simulink model "top10x20"  (Simulink 6.3)
settings: Solver=FixedStepDiscrete  StartTime=0.0  StopTime=3000  FixedStep=1  RelTol=1e-3
PreLoadFcn:
  | disp('Convolutional Interleaver 10x20')
  | disp(' 10 Branches')
  | disp(' FifoDepth = 20')
  | 
  | FifoDepth=20;
  | SymbolWidth = 8;
InitFcn:
  | %% DSPBuilder Start
  | alt_dspbuilder_update_model(bdroot)
  | %% DSPBuilder End
libraries: allblocks_alteradspbuilder2 x72, simulink x1
settings Model: LastModifiedBy=LKONG  StrictBusMsg=None
settings OptimizationCC: BooleanDataType=off  InlineInvariantSignals=on
settings DebuggingCC: SolverPrmCheckMsg=none
settings HardwareCC: TargetUnknown=on

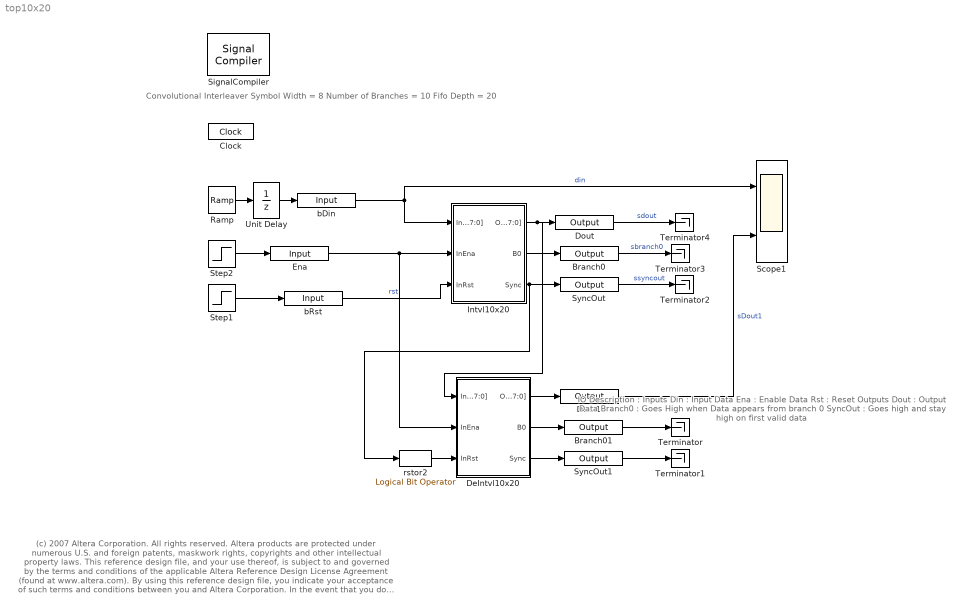
== system top10x20 ==
  note: (c) 2007 Altera Corporation. All rights reserved.  Altera products are protected under numerous U.S. and foreign patents, maskwork rights, copyrights and other intellectual property laws.
      | This reference design file, and your use thereof, is subject to and governed by the terms and conditions of the applicable Altera Reference Design License Agreement (found at www.altera.com).
      | By using this reference design file, you indicate your acceptance of such terms and conditions between you and Altera Corporation.
      | In the event that you do not agree with such terms and conditions, you may not use the reference design file and please promptly destroy any copies you have made.
      | This reference design file being provided on an "as-is" basis and as an accommodation and therefore all warranties, representations or guarantees of any kind (whether express, implied or statutory)
      | including, without limitation, warranties of merchantability, non-infringement, or fitness for a particular purpose, are specifically disclaimed.
      | By making this reference design file available, Altera expressly does not recommend, suggest or require that this reference design file be used in combination with any other product not provided by Altera
  note: IO Description :
      |
      | Inputs
      |            Din    : Input Data
      |            Ena   : Enable Data
      |            Rst    : Reset
      |
      | Outputs
      |           Dout        : Output Data
      |           Branch0 : Goes High when Data appears from branch 0
      |           SyncOut : Goes high and stay high on first valid data
  note: Convolutional Interleaver
      | Symbol Width = 8
      | Number of Branches = 10
      | Fifo Depth = 20
  Branch0 : allblocks_alteradspbuilder2/Output  iofile=d:\wsTrunk\workspace\Documentation\DesignExamples\Demos\Transforms\CrossInterleaver12x17\tb_top10x20\top10x20_Branch0.capture  BusType=Single Bit  bwl=1  bwr=0  PORTTYPE=Output
  Branch01 : allblocks_alteradspbuilder2/Output  iofile=d:\wsTrunk\workspace\Documentation\DesignExamples\Demos\Transforms\CrossInterleaver12x17\tb_top10x20\top10x20_Branch01.capture  BusType=Single Bit  bwl=1  bwr=0  PORTTYPE=Output
  Clock : allblocks_alteradspbuilder2/Clock  ClockPeriod=100  ClockPeriodUnit=ns  SampleTime=1  SimulationStartCycle=5  PhaseOffset=0  Reset=aclr  ResetType=Active Low  Export=off
  DeIntvl10x20 : Subsystem  AncestorBlock=ALTELINK/AltLab/HDL SubSystem
      mask Type: SubSystem AlteraBlockSet
  Dout : allblocks_alteradspbuilder2/Output  iofile=d:\wsTrunk\workspace\Documentation\DesignExamples\Demos\Transforms\CrossInterleaver12x17\tb_top10x20\top10x20_Dout.capture  BusType=Signed Integer  bwl=8  bwr=0  PORTTYPE=Output
  Dout1 : allblocks_alteradspbuilder2/Output  iofile=d:\wsTrunk\workspace\Documentation\DesignExamples\Demos\Transforms\CrossInterleaver12x17\tb_top10x20\top10x20_Dout1.capture  BusType=Signed Integer  bwl=8  bwr=0  PORTTYPE=Output
  Ena : allblocks_alteradspbuilder2/Input  iofile=d:\wsTrunk\workspace\Documentation\DesignExamples\Demos\Transforms\CrossInterleaver12x17\tb_top10x20\top10x20_Ena.salt  BusType=Single Bit  bwl=1  bwr=0  SpecifyClock=off  PORTTYPE=Input
  Intvl10x20 : Subsystem  AncestorBlock=ALTELINK/AltLab/HDL SubSystem
      mask Type: SubSystem AlteraBlockSet
  Ramp : simulink/Sources/Ramp  slope=1  start=0  X0=3
  Scope1 : Scope  NumInputPorts=2
      settings: YMin=-5~-5  YMax=5~5
  SignalCompiler : allblocks_alteradspbuilder2/Signal Compiler  DeviceFamily=Cyclone IV GX  DeviceName=AUTO  EnableSignalTap=off  SignalTapDepth=128  UseBoardBlock=off  StpUseDefaultClock=on  StpClock=Clock
  Step1 : Step  Time=3  Before=1  After=0  SampleTime=1
  Step2 : Step  SampleTime=1
  SyncOut : allblocks_alteradspbuilder2/Output  iofile=d:\wsTrunk\workspace\Documentation\DesignExamples\Demos\Transforms\CrossInterleaver12x17\tb_top10x20\top10x20_SyncOut.capture  BusType=Single Bit  bwl=1  bwr=0  PORTTYPE=Output
  SyncOut1 : allblocks_alteradspbuilder2/Output  iofile=d:\wsTrunk\workspace\Documentation\DesignExamples\Demos\Transforms\CrossInterleaver12x17\tb_top10x20\top10x20_SyncOut1.capture  BusType=Single Bit  bwl=1  bwr=0  PORTTYPE=Output
  Terminator{,1..4} (5 alike) : Terminator
  Unit Delay : UnitDelay
  bDin : allblocks_alteradspbuilder2/Input  iofile=d:\wsTrunk\workspace\Documentation\DesignExamples\Demos\Transforms\CrossInterleaver12x17\tb_top10x20\top10x20_bDin.salt  BusType=Signed Integer  bwl=8  bwr=0  SpecifyClock=off  PORTTYPE=Input
  bRst : allblocks_alteradspbuilder2/Input  iofile=d:\wsTrunk\workspace\Documentation\DesignExamples\Demos\Transforms\CrossInterleaver12x17\tb_top10x20\top10x20_bRst.salt  BusType=Single Bit  bwl=1  bwr=0  SpecifyClock=off  PORTTYPE=Input
  rstor2 : allblocks_alteradspbuilder2/Logical Bit Operator  LogicalOperator=NOT  user_inputs=2
  wires:
  Intvl10x20/1(Out1[7:0]) -> Dout/1, DeIntvl10x20/1(InDin[7:0])
  bDin/1 -> Scope1/1, Intvl10x20/1(InDin[7:0])  "din"
  Ena/1 -> DeIntvl10x20/2(InEna), Intvl10x20/2(InEna)
  bRst/1 -> Intvl10x20/3(InRst)  "rst"
  Ramp/1 -> Unit Delay/1
  Step1/1 -> bRst/1
  Step2/1 -> Ena/1
  Intvl10x20/2(B0) -> Branch0/1
  Intvl10x20/3(Sync) -> SyncOut/1, rstor2/1
  Unit Delay/1 -> bDin/1
  rstor2/1 -> DeIntvl10x20/3(InRst)
  DeIntvl10x20/1(Out1[7:0]) -> Dout1/1
  DeIntvl10x20/2(B0) -> Branch01/1
  DeIntvl10x20/3(Sync) -> SyncOut1/1
  Dout1/1 -> Scope1/2  "sDout1"
  Branch01/1 -> Terminator/1
  SyncOut1/1 -> Terminator1/1
  SyncOut/1 -> Terminator2/1  "ssyncout"
  Branch0/1 -> Terminator3/1  "sbranch0"
  Dout/1 -> Terminator4/1  "sdout"

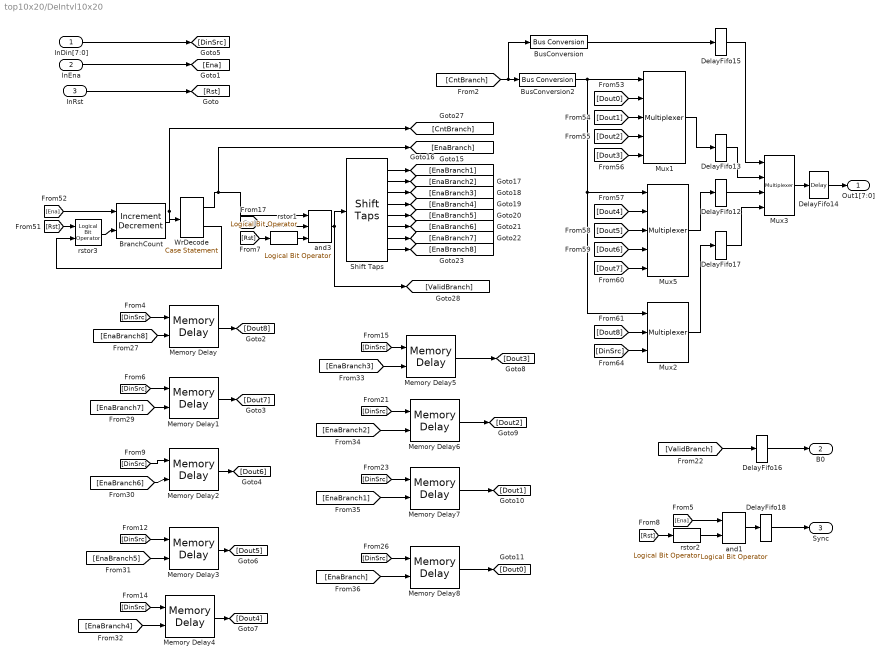
== system top10x20/DeIntvl10x20 ==
  InDin[7:0] : Inport
  InEna : Inport  Port=2
  InRst : Inport  Port=3
  BranchCount : allblocks_alteradspbuilder2/Increment Decrement  BusType=Unsigned Integer  bwl=4  bwr=0  SpecifyClock=off  clr_value=0  direction=Increment  phase_selection=1  use_ena=on  use_sclr=on
  BusConversion : allblocks_alteradspbuilder2/Bus Conversion  BusType=Unsigned Integer  ibwl=4  ibwr=0  bwl=2  bwr=0  bitToConnectToOutputLSB=2  round=off  saturate=off
  BusConversion2 : allblocks_alteradspbuilder2/Bus Conversion  BusType=Unsigned Integer  ibwl=4  ibwr=0  bwl=2  bwr=0  bitToConnectToOutputLSB=0  round=off  saturate=off
  DelayFifo{12..15,17} (5 alike) : allblocks_alteradspbuilder2/Delay  pipeline=1  ClockPhase=1  use_ena=off  use_sclr=off  use_init=off  reset_value=1
  DelayFifo16 : allblocks_alteradspbuilder2/Delay  pipeline=2  ClockPhase=1  use_ena=off  use_sclr=off  use_init=off  reset_value=1
  DelayFifo18 : allblocks_alteradspbuilder2/Delay  pipeline=2  ClockPhase=1  use_ena=off  use_sclr=off  use_init=off  reset_value=1
  Memory Delay : allblocks_alteradspbuilder2/Memory Delay  BusType=Inferred  bwl=8  bwr=0  pipeline=20  ram_type=AUTO  use_ena=on  use_sclr=off
  Memory Delay1 : allblocks_alteradspbuilder2/Memory Delay  BusType=Inferred  bwl=8  bwr=0  pipeline=40  ram_type=AUTO  use_ena=on  use_sclr=off
  Memory Delay2 : allblocks_alteradspbuilder2/Memory Delay  BusType=Inferred  bwl=8  bwr=0  pipeline=60  ram_type=AUTO  use_ena=on  use_sclr=off
  Memory Delay3 : allblocks_alteradspbuilder2/Memory Delay  BusType=Inferred  bwl=8  bwr=0  pipeline=80  ram_type=AUTO  use_ena=on  use_sclr=off
  Memory Delay4 : allblocks_alteradspbuilder2/Memory Delay  BusType=Inferred  bwl=8  bwr=0  pipeline=100  ram_type=AUTO  use_ena=on  use_sclr=off
  Memory Delay5 : allblocks_alteradspbuilder2/Memory Delay  BusType=Inferred  bwl=8  bwr=0  pipeline=120  ram_type=AUTO  use_ena=on  use_sclr=off
  Memory Delay6 : allblocks_alteradspbuilder2/Memory Delay  BusType=Inferred  bwl=8  bwr=0  pipeline=140  ram_type=AUTO  use_ena=on  use_sclr=off
  Memory Delay7 : allblocks_alteradspbuilder2/Memory Delay  BusType=Inferred  bwl=8  bwr=0  pipeline=160  ram_type=AUTO  use_ena=on  use_sclr=off
  Memory Delay8 : allblocks_alteradspbuilder2/Memory Delay  BusType=Inferred  bwl=8  bwr=0  pipeline=180  ram_type=AUTO  use_ena=on  use_sclr=off
  Mux1 : allblocks_alteradspbuilder2/Multiplexer  numInputs=4  pipeline=0  oneHot=off  use_ena=off  use_aclr=off
  Mux2 : allblocks_alteradspbuilder2/Multiplexer  numInputs=2  pipeline=0  oneHot=off  use_ena=off  use_aclr=off
  Mux3 : allblocks_alteradspbuilder2/Multiplexer  numInputs=3  pipeline=0  oneHot=off  use_ena=off  use_aclr=off
  Mux5 : allblocks_alteradspbuilder2/Multiplexer  numInputs=4  pipeline=0  oneHot=off  use_ena=off  use_aclr=off
  Shift Taps : allblocks_alteradspbuilder2/Shift Taps  number_of_taps=8  tap_distance=1  use_shiftout=off  use_ena=off  use_sclr=off  use_dedicated_circuitry=on  ram_type=AUTO
  WrDecode : allblocks_alteradspbuilder2/Case Statement  numOutputs=2  case_expression=0,9  formatted_case_expression=00000000,00001001  BusType=Signed Integer  bwl=8  bwr=0  pipeline=off  hasDefault=off
  and1 : allblocks_alteradspbuilder2/Logical Bit Operator  LogicalOperator=AND  user_inputs=2
  and3 : allblocks_alteradspbuilder2/Logical Bit Operator  LogicalOperator=AND  user_inputs=3
  rstor1 : allblocks_alteradspbuilder2/Logical Bit Operator  LogicalOperator=NOT  user_inputs=2
  rstor2 : allblocks_alteradspbuilder2/Logical Bit Operator  LogicalOperator=NOT  user_inputs=2
  rstor3 : allblocks_alteradspbuilder2/Logical Bit Operator  LogicalOperator=OR  user_inputs=2
  Out1[7:0] : Outport
  B0 : Outport  Port=2
  Sync : Outport  Port=3
  wires:
  and1/1 -> DelayFifo18/1
  rstor2/1 -> and1/2
  [Ena] -> and1/1
  [Rst] -> rstor2/1
  DelayFifo18/1 -> Sync/1
  BusConversion2/1 -> Mux2/1, Mux5/1, Mux1/1
  [CntBranch] -> BusConversion/1, BusConversion2/1
  Mux2/1 -> DelayFifo17/1
  Mux5/1 -> DelayFifo12/1
  DelayFifo17/1 -> Mux3/4
  DelayFifo12/1 -> Mux3/3
  Mux1/1 -> DelayFifo13/1
  DelayFifo16/1 -> B0/1
  [ValidBranch] -> DelayFifo16/1
  rstor1/1 -> and3/3
  [Ena] -> and3/2
  [Rst] -> rstor1/1
  and3/1 -> [ValidBranch], Shift Taps/1
  DelayFifo15/1 -> Mux3/1
  WrDecode/1 -> and3/1, [EnaBranch]
  DelayFifo13/1 -> Mux3/2
  [DinSrc] -> Mux2/3
  [Dout8] -> Mux2/2
  [Dout7] -> Mux5/5
  [Dout6] -> Mux5/4
  [Dout5] -> Mux5/3
  [Dout4] -> Mux5/2
  [Dout3] -> Mux1/5
  [Dout2] -> Mux1/4
  [Dout1] -> Mux1/3
  [Dout0] -> Mux1/2
  BusConversion/1 -> DelayFifo15/1
  Mux3/1 -> DelayFifo14/1
  Shift Taps/1 -> [EnaBranch1]
  Shift Taps/2 -> [EnaBranch2]
  Shift Taps/3 -> [EnaBranch3]
  Shift Taps/4 -> [EnaBranch4]
  Shift Taps/5 -> [EnaBranch5]
  Shift Taps/6 -> [EnaBranch6]
  Shift Taps/7 -> [EnaBranch7]
  Shift Taps/8 -> [EnaBranch8]
  [Ena] -> BranchCount/1
  [Rst] -> rstor3/1
  rstor3/1 -> BranchCount/2
  WrDecode/2 -> rstor3/2
  BranchCount/1 -> WrDecode/1, [CntBranch]
  DelayFifo14/1 -> Out1[7:0]/1
  [EnaBranch2] -> Memory Delay6/2
  [EnaBranch1] -> Memory Delay7/2
  [EnaBranch] -> Memory Delay8/2
  [EnaBranch3] -> Memory Delay5/2
  [EnaBranch4] -> Memory Delay4/2
  [EnaBranch5] -> Memory Delay3/2
  [EnaBranch6] -> Memory Delay2/2
  [EnaBranch7] -> Memory Delay1/2
  [EnaBranch8] -> Memory Delay/2
  Memory Delay8/1 -> [Dout0]
  Memory Delay7/1 -> [Dout1]
  Memory Delay6/1 -> [Dout2]
  Memory Delay5/1 -> [Dout3]
  Memory Delay4/1 -> [Dout4]
  Memory Delay3/1 -> [Dout5]
  Memory Delay2/1 -> [Dout6]
  Memory Delay1/1 -> [Dout7]
  Memory Delay/1 -> [Dout8]
  [DinSrc] -> Memory Delay8/1
  [DinSrc] -> Memory Delay7/1
  [DinSrc] -> Memory Delay6/1
  [DinSrc] -> Memory Delay5/1
  [DinSrc] -> Memory Delay4/1
  [DinSrc] -> Memory Delay3/1
  [DinSrc] -> Memory Delay2/1
  [DinSrc] -> Memory Delay1/1
  [DinSrc] -> Memory Delay/1
  InRst/1 -> [Rst]
  InEna/1 -> [Ena]
  InDin[7:0]/1 -> [DinSrc]

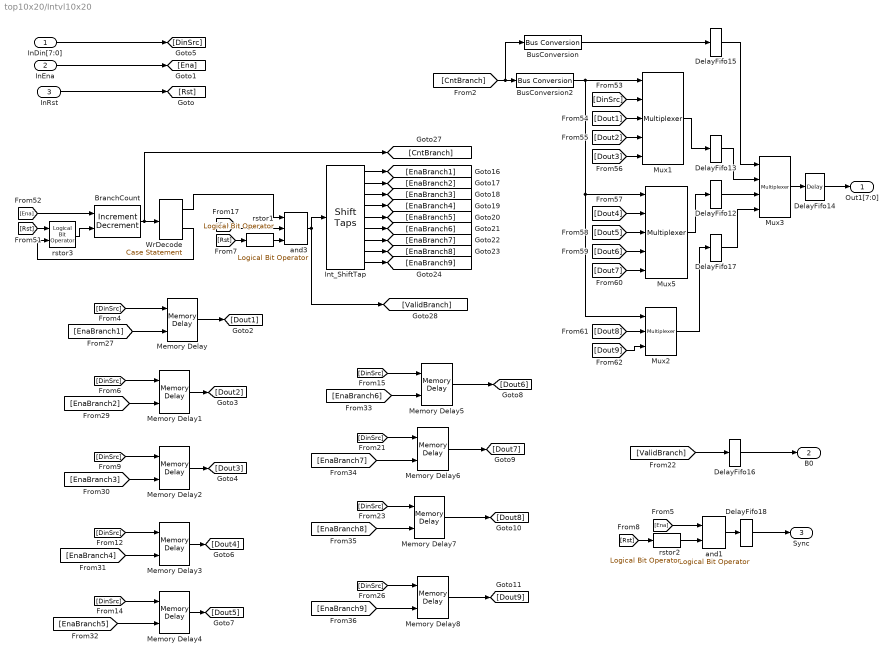
== system top10x20/Intvl10x20 ==
  InDin[7:0] : Inport
  InEna : Inport  Port=2
  InRst : Inport  Port=3
  BranchCount : allblocks_alteradspbuilder2/Increment Decrement  BusType=Unsigned Integer  bwl=4  bwr=0  SpecifyClock=off  clr_value=0  direction=Increment  phase_selection=1  use_ena=on  use_sclr=on
  BusConversion : allblocks_alteradspbuilder2/Bus Conversion  BusType=Unsigned Integer  ibwl=4  ibwr=0  bwl=2  bwr=0  bitToConnectToOutputLSB=2  round=off  saturate=off
  BusConversion2 : allblocks_alteradspbuilder2/Bus Conversion  BusType=Unsigned Integer  ibwl=4  ibwr=0  bwl=2  bwr=0  bitToConnectToOutputLSB=0  round=off  saturate=off
  DelayFifo{12..15,17} (5 alike) : allblocks_alteradspbuilder2/Delay  pipeline=1  ClockPhase=1  use_ena=off  use_sclr=off  use_init=off  reset_value=1
  DelayFifo16 : allblocks_alteradspbuilder2/Delay  pipeline=2  ClockPhase=1  use_ena=off  use_sclr=off  use_init=off  reset_value=1
  DelayFifo18 : allblocks_alteradspbuilder2/Delay  pipeline=2  ClockPhase=1  use_ena=off  use_sclr=off  use_init=off  reset_value=1
  Int_ShiftTap : allblocks_alteradspbuilder2/Shift Taps  number_of_taps=9  tap_distance=1  use_shiftout=off  use_ena=off  use_sclr=off  use_dedicated_circuitry=on  ram_type=AUTO
  Memory Delay : allblocks_alteradspbuilder2/Memory Delay  BusType=Inferred  bwl=8  bwr=0  pipeline=20  ram_type=AUTO  use_ena=on  use_sclr=off
  Memory Delay1 : allblocks_alteradspbuilder2/Memory Delay  BusType=Inferred  bwl=8  bwr=0  pipeline=40  ram_type=AUTO  use_ena=on  use_sclr=off
  Memory Delay2 : allblocks_alteradspbuilder2/Memory Delay  BusType=Inferred  bwl=8  bwr=0  pipeline=60  ram_type=AUTO  use_ena=on  use_sclr=off
  Memory Delay3 : allblocks_alteradspbuilder2/Memory Delay  BusType=Inferred  bwl=8  bwr=0  pipeline=80  ram_type=AUTO  use_ena=on  use_sclr=off
  Memory Delay4 : allblocks_alteradspbuilder2/Memory Delay  BusType=Inferred  bwl=8  bwr=0  pipeline=100  ram_type=AUTO  use_ena=on  use_sclr=off
  Memory Delay5 : allblocks_alteradspbuilder2/Memory Delay  BusType=Inferred  bwl=8  bwr=0  pipeline=120  ram_type=AUTO  use_ena=on  use_sclr=off
  Memory Delay6 : allblocks_alteradspbuilder2/Memory Delay  BusType=Inferred  bwl=8  bwr=0  pipeline=140  ram_type=AUTO  use_ena=on  use_sclr=off
  Memory Delay7 : allblocks_alteradspbuilder2/Memory Delay  BusType=Inferred  bwl=8  bwr=0  pipeline=160  ram_type=AUTO  use_ena=on  use_sclr=off
  Memory Delay8 : allblocks_alteradspbuilder2/Memory Delay  BusType=Inferred  bwl=8  bwr=0  pipeline=180  ram_type=AUTO  use_ena=on  use_sclr=off
  Mux1 : allblocks_alteradspbuilder2/Multiplexer  numInputs=4  pipeline=0  oneHot=off  use_ena=off  use_aclr=off
  Mux2 : allblocks_alteradspbuilder2/Multiplexer  numInputs=2  pipeline=0  oneHot=off  use_ena=off  use_aclr=off
  Mux3 : allblocks_alteradspbuilder2/Multiplexer  numInputs=3  pipeline=0  oneHot=off  use_ena=off  use_aclr=off
  Mux5 : allblocks_alteradspbuilder2/Multiplexer  numInputs=4  pipeline=0  oneHot=off  use_ena=off  use_aclr=off
  WrDecode : allblocks_alteradspbuilder2/Case Statement  numOutputs=2  case_expression=0,9  formatted_case_expression=00000000,00001001  BusType=Signed Integer  bwl=8  bwr=0  pipeline=off  hasDefault=off
  and1 : allblocks_alteradspbuilder2/Logical Bit Operator  LogicalOperator=AND  user_inputs=2
  and3 : allblocks_alteradspbuilder2/Logical Bit Operator  LogicalOperator=AND  user_inputs=3
  rstor1 : allblocks_alteradspbuilder2/Logical Bit Operator  LogicalOperator=NOT  user_inputs=2
  rstor2 : allblocks_alteradspbuilder2/Logical Bit Operator  LogicalOperator=NOT  user_inputs=2
  rstor3 : allblocks_alteradspbuilder2/Logical Bit Operator  LogicalOperator=OR  user_inputs=2
  Out1[7:0] : Outport
  B0 : Outport  Port=2
  Sync : Outport  Port=3
  wires:
  and1/1 -> DelayFifo18/1
  rstor2/1 -> and1/2
  [Ena] -> and1/1
  [Rst] -> rstor2/1
  DelayFifo18/1 -> Sync/1
  BusConversion2/1 -> Mux2/1, Mux5/1, Mux1/1
  [CntBranch] -> BusConversion/1, BusConversion2/1
  Mux2/1 -> DelayFifo17/1
  Mux5/1 -> DelayFifo12/1
  DelayFifo17/1 -> Mux3/4
  DelayFifo12/1 -> Mux3/3
  Mux1/1 -> DelayFifo13/1
  DelayFifo16/1 -> B0/1
  [ValidBranch] -> DelayFifo16/1
  rstor1/1 -> and3/3
  [Ena] -> and3/2
  [Rst] -> rstor1/1
  and3/1 -> [ValidBranch], Int_ShiftTap/1
  DelayFifo15/1 -> Mux3/1
  WrDecode/1 -> and3/1
  DelayFifo13/1 -> Mux3/2
  [Dout9] -> Mux2/3
  [Dout8] -> Mux2/2
  [Dout7] -> Mux5/5
  [Dout6] -> Mux5/4
  [Dout5] -> Mux5/3
  [Dout4] -> Mux5/2
  [Dout3] -> Mux1/5
  [Dout2] -> Mux1/4
  [Dout1] -> Mux1/3
  [DinSrc] -> Mux1/2
  BusConversion/1 -> DelayFifo15/1
  Mux3/1 -> DelayFifo14/1
  Int_ShiftTap/1 -> [EnaBranch1]
  Int_ShiftTap/2 -> [EnaBranch2]
  Int_ShiftTap/3 -> [EnaBranch3]
  Int_ShiftTap/4 -> [EnaBranch4]
  Int_ShiftTap/5 -> [EnaBranch5]
  Int_ShiftTap/6 -> [EnaBranch6]
  Int_ShiftTap/7 -> [EnaBranch7]
  Int_ShiftTap/8 -> [EnaBranch8]
  Int_ShiftTap/9 -> [EnaBranch9]
  [Ena] -> BranchCount/1
  [Rst] -> rstor3/1
  rstor3/1 -> BranchCount/2
  WrDecode/2 -> rstor3/2
  BranchCount/1 -> [CntBranch], WrDecode/1
  DelayFifo14/1 -> Out1[7:0]/1
  [EnaBranch7] -> Memory Delay6/2
  [EnaBranch8] -> Memory Delay7/2
  [EnaBranch9] -> Memory Delay8/2
  [EnaBranch6] -> Memory Delay5/2
  [EnaBranch5] -> Memory Delay4/2
  [EnaBranch4] -> Memory Delay3/2
  [EnaBranch3] -> Memory Delay2/2
  [EnaBranch2] -> Memory Delay1/2
  [EnaBranch1] -> Memory Delay/2
  Memory Delay8/1 -> [Dout9]
  Memory Delay7/1 -> [Dout8]
  Memory Delay6/1 -> [Dout7]
  Memory Delay5/1 -> [Dout6]
  Memory Delay4/1 -> [Dout5]
  Memory Delay3/1 -> [Dout4]
  Memory Delay2/1 -> [Dout3]
  Memory Delay1/1 -> [Dout2]
  Memory Delay/1 -> [Dout1]
  [DinSrc] -> Memory Delay8/1
  [DinSrc] -> Memory Delay7/1
  [DinSrc] -> Memory Delay6/1
  [DinSrc] -> Memory Delay5/1
  [DinSrc] -> Memory Delay4/1
  [DinSrc] -> Memory Delay3/1
  [DinSrc] -> Memory Delay2/1
  [DinSrc] -> Memory Delay1/1
  [DinSrc] -> Memory Delay/1
  InRst/1 -> [Rst]
  InEna/1 -> [Ena]
  InDin[7:0]/1 -> [DinSrc]
